simulink model "gm_pulse_detector_v4"  (R2022b)
settings: Solver=FixedStepDiscrete  StartTime=0.0  StopTime=SimTime  RelTol=1e-3
undefined symbols (not defined in the file or in its folder): CorrFilter, threshold, WindowLen
libraries: dspsrcs4 x2, dsphdlfiltering2 x1, simulink x1, hdlsllib x1
settings Model: Creator=Lenovo  LastModifiedBy=Lenovo
settings OptimizationCC: BlockReduction=off  ConditionallyExecuteInputs=off  DefaultParameterBehavior=Inlined  InheritOutputTypeSmallerThanSingle=on
settings DebuggingCC: AlgebraicLoopMsg=error  InheritedTsInSrcMsg=none  SingleTaskRateTransMsg=error
settings HardwareCC: ProdBitPerPointer=32  ProdBitPerSizeT=32  ProdBitPerPtrDiffT=32  ProdLargestAtomicFloat=None  ProdIntDivRoundTo=Undefined  ProdEndianess=Unspecified  ProdWordSize=32  ProdHWDeviceType=ASIC/FPGA->ASIC/FPGA  TargetBitPerPointer=64  TargetBitPerSizeT=64  TargetBitPerPtrDiffT=64  TargetLongLongMode=on  TargetIntDivRoundTo=Zero  TargetEndianess=LittleEndian  TargetWordSize=64  TargetHWDeviceType=Custom Processor->MATLAB Host Computer  ProdEqTarget=off

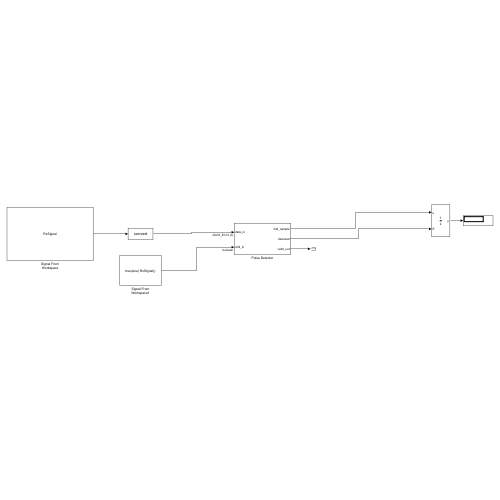
[thumbnail: Simulink's stored preview of the top-level diagram]
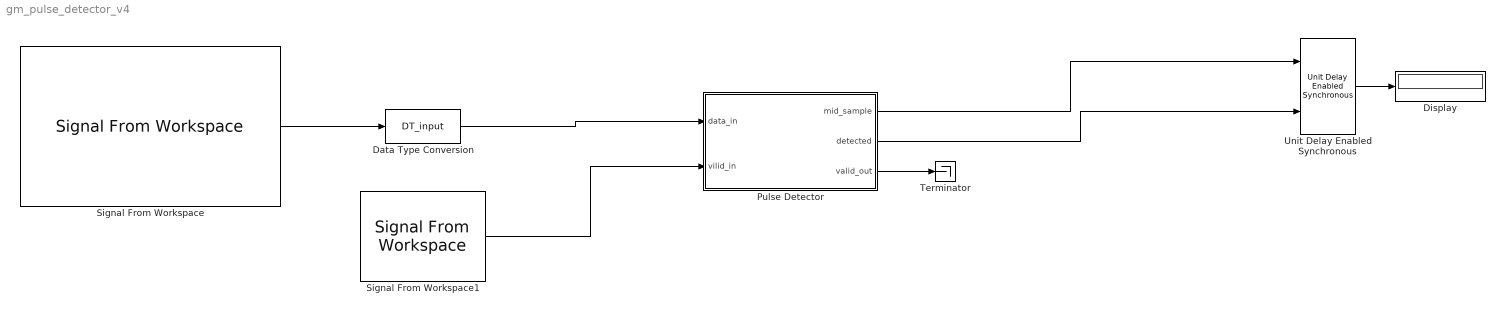
== system gm_pulse_detector_v4 ==
  Data Type Conversion : DataTypeConversion  OutDataTypeStr=DT_input  SaturateOnIntegerOverflow=off  RndMeth=Floor
  Display : Display
  Pulse Detector : Subsystem
  Signal From Workspace : dspsrcs4/Signal From Workspace  X=RxSignal  Ts=1  nsamps=1  OutputAfterFinalValue=Setting to zero  ignoreOrWarnInputAndFrameLengths=off  OutputFrames=off
  Signal From Workspace1 : dspsrcs4/Signal From Workspace  X=true(size( RxSignal))  Ts=1  nsamps=1  OutputAfterFinalValue=Setting to zero  ignoreOrWarnInputAndFrameLengths=off  OutputFrames=off
  Terminator : Terminator
  Unit Delay Enabled Synchronous : hdlsllib/Discrete/Unit Delay Enabled Synchronous  InitialCondition=0.0  SampleTime=-1
  wires:
  Data Type Conversion/1 -> Pulse Detector/1(data_in)
  Pulse Detector/3(valid_out) -> Terminator/1
  Signal From Workspace1/1 -> Pulse Detector/2(vilid_in)
  Pulse Detector/2(detected) -> Unit Delay Enabled Synchronous/2
  Pulse Detector/1(mid_sample) -> Unit Delay Enabled Synchronous/1
  Signal From Workspace/1 -> Data Type Conversion/1
  Unit Delay Enabled Synchronous/1 -> Display/1

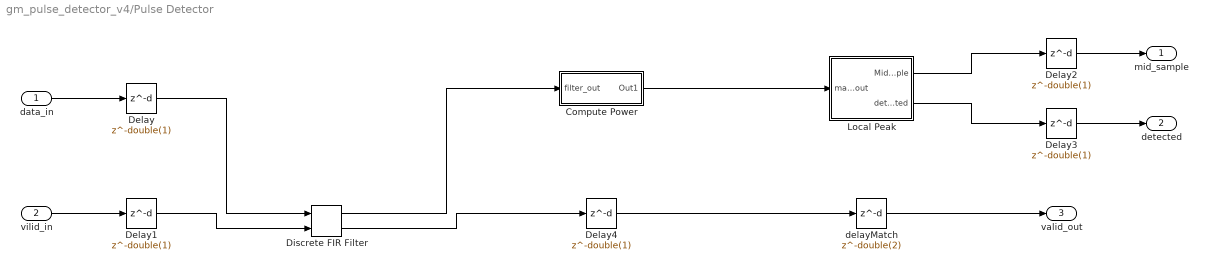
== system gm_pulse_detector_v4/Pulse Detector ==
  data_in : Inport  OutDataTypeStr=fixdt(1, 16, 14)  PortDimensions=1  SampleTime=1
      settings: SignalType=complex
  vilid_in : Inport  Port=2  OutDataTypeStr=boolean  PortDimensions=1  SampleTime=1
  Compute Power : Subsystem
  Delay{,1..4} (5 alike) : Delay  DelayLength=double(1)  InitialCondition=0  SampleTime=1
  Discrete FIR Filter : dsphdlfiltering2/Discrete FIR Filter  NumeratorSource=Property  Numerator=CorrFilter  NumeratorPrototype=[]  FilterStructure=Direct form systolic  SerializationOption=Minimum number of cycles between valid input samples  NumCycles=2  NumberOfMultipliers=2  SimulateUsing=Code generation  roundingMode=Floor  overflowMode=off  CoefficientsDataTypeStr=DT_coeff  ResetInputPort=off  HDLGlobalReset=off
  Local Peak : Subsystem
  delayMatch : Delay  DelayLength=double(2)  InitialCondition=0  SampleTime=1
  mid_sample : Outport  SampleTime=1
  detected : Outport  Port=2  SampleTime=1
  valid_out : Outport  Port=3  SampleTime=1
  wires:
  data_in/1 -> Delay/1
  vilid_in/1 -> Delay1/1
  Compute Power/1(Out1) -> Local Peak/1(mag_sq_out)
  Delay/1 -> Discrete FIR Filter/1
  Delay1/1 -> Discrete FIR Filter/2
  Delay2/1 -> mid_sample/1
  Delay3/1 -> detected/1
  delayMatch/1 -> valid_out/1
  Discrete FIR Filter/1 -> Compute Power/1(filter_out)
  Discrete FIR Filter/2 -> Delay4/1
  Local Peak/1(MidSample) -> Delay2/1
  Local Peak/2(detected) -> Delay3/1
  Delay4/1 -> delayMatch/1

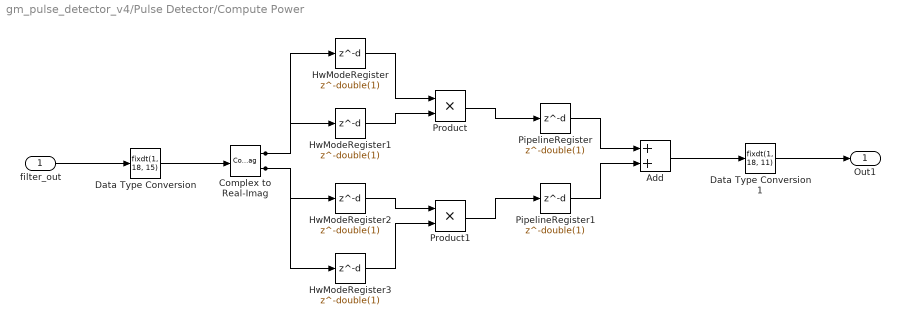
== system gm_pulse_detector_v4/Pulse Detector/Compute Power ==
  filter_out : Inport  OutDataTypeStr=fixdt(1, 40, 37)  PortDimensions=1  SampleTime=1
      settings: SignalType=complex
  Add : Sum  AccumDataTypeStr=fixdt(1, 37, 30)  OutDataTypeStr=fixdt(1, 37, 30)  SampleTime=1
  Complex to Real-Imag : ComplexToRealImag  SampleTime=1
  Data Type Conversion : DataTypeConversion  OutDataTypeStr=fixdt(1, 18, 15)  SampleTime=1  SaturateOnIntegerOverflow=off  RndMeth=Floor
  Data Type Conversion1 : DataTypeConversion  OutDataTypeStr=fixdt(1, 18, 11)  SampleTime=1  SaturateOnIntegerOverflow=off  RndMeth=Floor
  HwModeRegister{,1..3} (4 alike) : Delay  DelayLength=double(1)  InitialCondition=0  SampleTime=1
  PipelineRegister : Delay  DelayLength=double(1)  InitialCondition=0  SampleTime=1
  PipelineRegister1 : Delay  DelayLength=double(1)  InitialCondition=0  SampleTime=1
  Product : Product  Inputs=**  OutDataTypeStr=fixdt(1, 36, 30)  SampleTime=1
  Product1 : Product  Inputs=**  OutDataTypeStr=fixdt(1, 36, 30)  SampleTime=1
  Out1 : Outport  SampleTime=1
  wires:
  Add/1 -> Data Type Conversion1/1
  Complex to Real-Imag/1 -> HwModeRegister/1, HwModeRegister1/1
  Complex to Real-Imag/2 -> HwModeRegister2/1, HwModeRegister3/1
  Data Type Conversion/1 -> Complex to Real-Imag/1
  Data Type Conversion1/1 -> Out1/1
  PipelineRegister/1 -> Add/1
  PipelineRegister1/1 -> Add/2
  filter_out/1 -> Data Type Conversion/1
  Product/1 -> PipelineRegister/1
  HwModeRegister/1 -> Product/1
  HwModeRegister1/1 -> Product/2
  Product1/1 -> PipelineRegister1/1
  HwModeRegister2/1 -> Product1/1
  HwModeRegister3/1 -> Product1/2

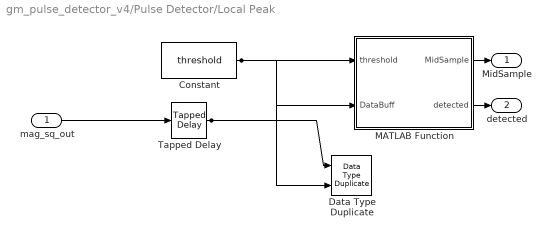
== system gm_pulse_detector_v4/Pulse Detector/Local Peak ==
  mag_sq_out : Inport  OutDataTypeStr=fixdt(1, 18, 11)  PortDimensions=1  SampleTime=1
  Constant : Constant  Value=threshold  OutDataTypeStr=Inherit: Inherit via back propagation  SampleTime=-1
  Data Type Duplicate : DataTypeDuplicate
  MATLAB Function : Subsystem
  Tapped Delay : simulink/Discrete/Tapped Delay  vinit=0.0  samptime=-1  NumDelays=WindowLen  DelayOrder=Oldest  includeCurrent=off
  MidSample : Outport  SampleTime=1
  detected : Outport  Port=2  SampleTime=1
  wires:
  Constant/1 -> Data Type Duplicate/2, MATLAB Function/1(threshold)
  MATLAB Function/1(MidSample) -> MidSample/1
  MATLAB Function/2(detected) -> detected/1
  Tapped Delay/1 -> Data Type Duplicate/1, MATLAB Function/2(DataBuff)
  mag_sq_out/1 -> Tapped Delay/1

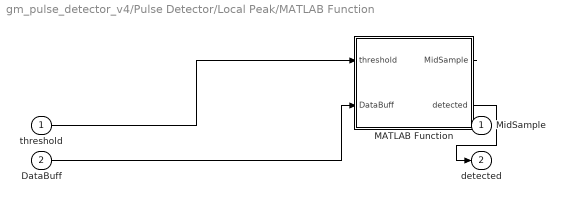
== system gm_pulse_detector_v4/Pulse Detector/Local Peak/MATLAB Function ==
  threshold : Inport  OutDataTypeStr=fixdt(1, 18, 11)  PortDimensions=1  SampleTime=1
  DataBuff : Inport  Port=2  OutDataTypeStr=fixdt(1, 18, 11)  PortDimensions=[11]  SampleTime=1
  MATLAB Function : MATLAB Function  TreatAsAtomicUnit=on
  MidSample : Outport  SampleTime=1
  detected : Outport  Port=2  SampleTime=1
  wires:
  MATLAB Function/1(MidSample) -> MidSample/1
  MATLAB Function/2(detected) -> detected/1
  threshold/1 -> MATLAB Function/1(threshold)
  DataBuff/1 -> MATLAB Function/2(DataBuff)

== matlab function gm_pulse_detector_v4/Pulse Detector/Local Peak/MATLAB Function/MATLAB Function ==
  settings: fimath=fimath('RoundingMethod', 'Floor','OverflowAction', 'Wrap','ProductMode', 'FullPrecision', 'SumMode', 'FullPrecision')
  data: MidSample output; threshold input; DataBuff input; detected output; WindowLen parameter
function [MidSample,detected]=fcn(threshold,DataBuff, WindowLen)

MidIdx = ceil(WindowLen/2);

MidSample=DataBuff(MidIdx);
CompareOut=DataBuff-MidSample;



    % if all values in the result are negative and the middle sample is
    % greater than a threshold, it is a local max
if all(CompareOut <= 0) && (MidSample > threshold)
    detected=true;
else
    detected=false;
end
